simulink model "contactCheck"  (R2023a)
settings: Solver=FixedStepAuto  StartTime=0.0  StopTime=inf  RelTol=1e-3
libraries: mjLib x1
settings Model: Creator=vmano  LastModifiedBy=mvelmuru
settings OptimizationCC: ReuseModelBlockBuffer=off

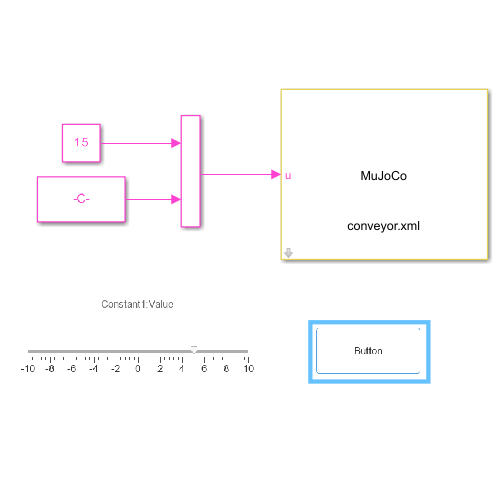
[thumbnail: Simulink's stored preview of the top-level diagram]
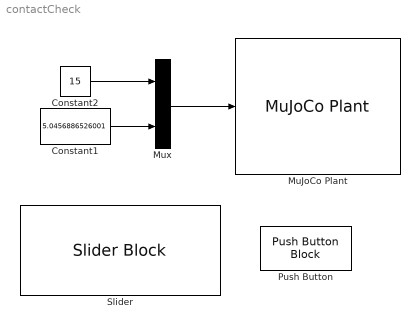
== system contactCheck ==
  Constant1 : Constant  Value=5.0456886526001
  Constant2 : Constant  Value=15
  MuJoCo Plant : mjLib/MuJoCo Plant  controlBus=[]  sensorBus=mj_bus_sensor_7979902499018342666  controlLength=[]  sensorLength=[]  rgbLength=[]  depthLength=[]  sampleTime=0.002  xmlFileRel=./models/conveyor.xml  xmlFile=./models/conveyor.xml  renderingType=Global  vsync=off  visualFPS=60  zoomLevel=1  znear=0.03  zfar=150  cameraSampleTime=0.020  rgbOutOption=on  depthOutOption=on  controlInterfaceType=Vector
      settings: SourceProductName=MuJoCo Simulator
  Mux : Mux  Inputs=2
  Push Button : PushButtonBlock  OnValue=-15  ButtonType=Latch  OffValue=15.000000
  Slider : SliderBlock  ScaleMin=-10  ScaleMax=10
  wires:
  Mux/1 -> MuJoCo Plant/1
  Constant2/1 -> Mux/1
  Constant1/1 -> Mux/2
